simulink model "massign"  (Simulink 6.3)
settings: Solver=ode1  StartTime=0.0  StopTime=1  FixedStep=1  RelTol=1e-3
settings Model: Creator=mtocci  LastModifiedBy=mshakeri  ExtModeAutoUpdateStatusClock=off  StrictBusMsg=ErrorLevel1
settings DataIOCC: SignalLoggingName=logsOut
settings OptimizationCC: BooleanDataType=off  InlineParams=on  InlineInvariantSignals=on
settings DebuggingCC: SolverPrmCheckMsg=none

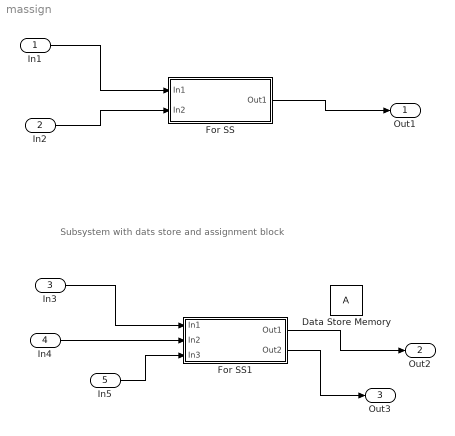
== system massign ==
  note: Subsystem with dats store and assignment block
  In1 : Inport  Port=1  LatchInput=off
  In2 : Inport  Port=2  LatchInput=off
  In3 : Inport  Port=3  LatchInput=off
  In4 : Inport  Port=4  LatchInput=off
  In5 : Inport  Port=5  LatchInput=off
  Data Store Memory : DataStoreMemory  DataStoreName=A  ReadBeforeWriteMsg=warning  WriteAfterWriteMsg=warning  WriteAfterReadMsg=warning  InitialValue=0
  For SS : Subsystem  TreatAsAtomicUnit=on
  For SS1 : Subsystem  TreatAsAtomicUnit=on
  Out1 : Outport
  Out2 : Outport  Port=2
  Out3 : Outport  Port=3
  wires:
  In1/1 -> For SS/1(In1)
  For SS/1(Out1) -> Out1/1
  In2/1 -> For SS/2(In2)
  In3/1 -> For SS1/1(In1)
  For SS1/1(Out1) -> Out2/1
  In4/1 -> For SS1/2(In2)
  In5/1 -> For SS1/3(In3)
  For SS1/2(Out2) -> Out3/1

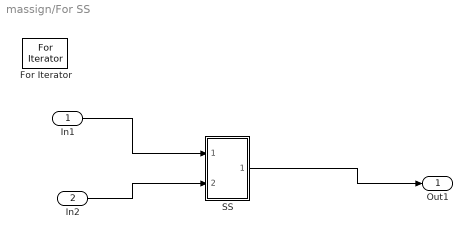
== system massign/For SS ==
  In1 : Inport  Port=1  LatchInput=off
  In2 : Inport  Port=2  LatchInput=off
  For Iterator : ForIterator  ShowIterationPort=off
  SS : Subsystem  TreatAsAtomicUnit=on
  Out1 : Outport
  wires:
  In1/1 -> SS/1(In1)
  SS/1(Out1) -> Out1/1
  In2/1 -> SS/2(In2)

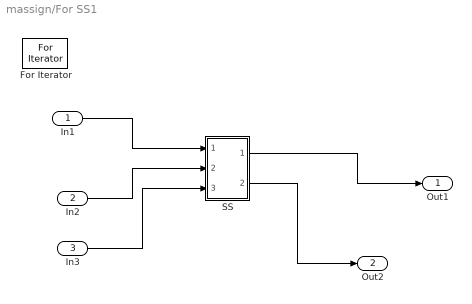
== system massign/For SS1 ==
  In1 : Inport  Port=1  LatchInput=off
  In2 : Inport  Port=2  LatchInput=off
  In3 : Inport  Port=3  LatchInput=off
  For Iterator : ForIterator  ShowIterationPort=off
  SS : Subsystem  TreatAsAtomicUnit=on
  Out1 : Outport
  Out2 : Outport  Port=2
  wires:
  In2/1 -> SS/2(In2)
  SS/1(Out1) -> Out1/1
  In1/1 -> SS/1(In1)
  In3/1 -> SS/3(In3)
  SS/2(Out2) -> Out2/1

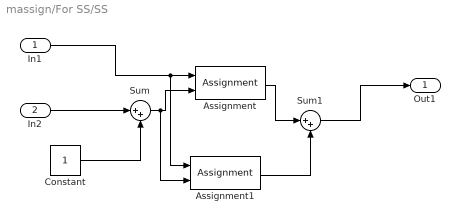
== system massign/For SS/SS ==
  In1 : Inport  Port=1  PortDimensions=5  LatchInput=off
  In2 : Inport  Port=2  PortDimensions=1  LatchInput=off
  Assignment : Assignment  DiagnosticForDimensions=Error
  Assignment1 : Assignment  DiagnosticForDimensions=Error
  Constant : Constant
  Sum : Sum  Inputs=|++
  Sum1 : Sum  Inputs=|++
  Out1 : Outport
  wires:
  Sum1/1 -> Out1/1
  Assignment1/1 -> Sum1/2
  Assignment/1 -> Sum1/1
  In2/1 -> Sum/1
  Sum/1 -> Assignment1/2, Assignment/2
  In1/1 -> Assignment1/1, Assignment/1
  Constant/1 -> Sum/2

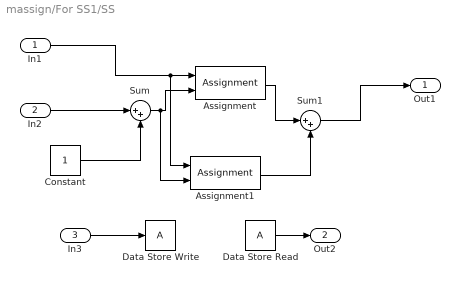
== system massign/For SS1/SS ==
  In1 : Inport  Port=1  PortDimensions=5  LatchInput=off
  In2 : Inport  Port=2  PortDimensions=1  LatchInput=off
  In3 : Inport  Port=3  LatchInput=off
  Assignment : Assignment  DiagnosticForDimensions=Error
  Assignment1 : Assignment  DiagnosticForDimensions=Error
  Constant : Constant
  Data Store Read : DataStoreRead  DataStoreName=A  SampleTime=-1
  Data Store Write : DataStoreWrite  DataStoreName=A  SampleTime=-1
  Sum : Sum  Inputs=|++
  Sum1 : Sum  Inputs=|++
  Out1 : Outport
  Out2 : Outport  Port=2
  wires:
  Constant/1 -> Sum/2
  In1/1 -> Assignment/1, Assignment1/1
  Sum/1 -> Assignment/2, Assignment1/2
  In2/1 -> Sum/1
  Assignment/1 -> Sum1/1
  Assignment1/1 -> Sum1/2
  Sum1/1 -> Out1/1
  In3/1 -> Data Store Write/1
  Data Store Read/1 -> Out2/1
